simulink model "Car"  (R2023a)
settings: Solver=VariableStepAuto  StartTime=0.0  StopTime=1000  RelTol=1e-3
values from neighbouring files (symbols this model uses):
  AIR_DENSITY = 1.2    [Setup.m]
  FRONTAL_AREA = 1    [Setup.m]
  FULL_PACK_KWH = HV_PACK_VOLTAGE * HV_PACK_CAPACITY * UNIT_TO_KILO    (= 7.68)    [Setup.m]
  HV_PACK_VOLTAGE = 96    [Setup.m]
  INT_CURRENTS = CURRENT_DATA_ECO(1):0.0001:CURRENT_DATA_ECO(end)    [Setup.m]
  INT_TORQUES_ECO = interp1(CURRENT_DATA_ECO, TORQUES_DATA_ECO, INTERMEDIATE_VALUES,'spline')    [Setup.m]
  STARTING_KWH = FULL_PACK_KWH * (1 - 0.00)    (= 7.68)    [Setup.m]
  TARGET_SPEED = 25    [Setup.m]
  TOTAL_MASS = CAR_MASS + DRIVER_MASS    (= 282.996279643)    [Setup.m]
  UNIT_TO_KILO = 1 / 1000    (= 0.001)    [Setup.m]
undefined symbols (not defined in the file or in its folder): C_ROLLING_RESISTANCE, GRAVITY, MAX_TORQUE, WHEEL_RADIUS
libraries: slpidlib x1, simulink x1
settings Model: Creator=jcpetrie  LastModifiedBy=jcpetrie
settings ModelReferenceCC: EnableRefExpFcnMdlSchedulingChecks=on

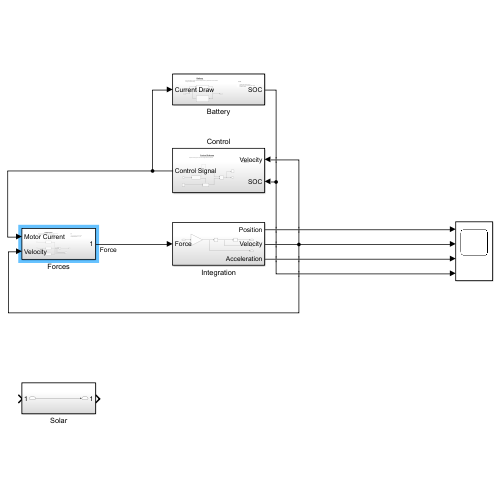
[thumbnail: Simulink's stored preview of the top-level diagram]
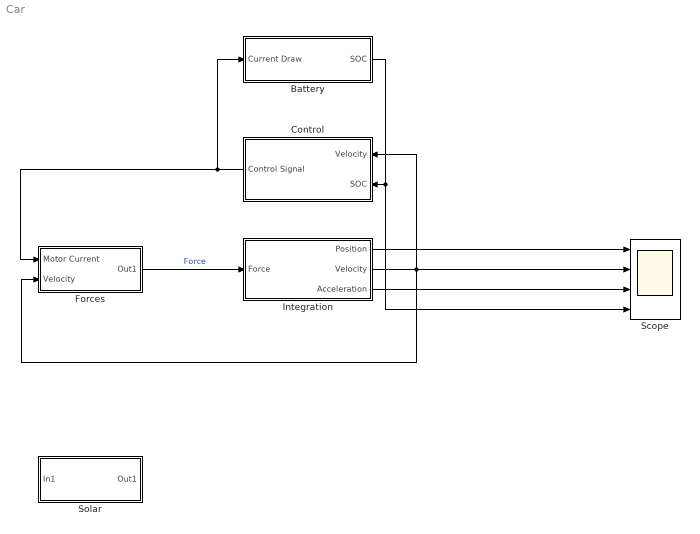
== system Car ==
  Battery : Subsystem
  Control : Subsystem
  Forces : Subsystem
  Integration : Subsystem
  Scope : Scope  NumInputPorts=4
  Solar : Subsystem
  wires:
  Control/1(Control Signal) -> Battery/1(Current Draw), Forces/1(Motor Current)
  Integration/2(Velocity) -> Forces/2(Velocity), Scope/2, Control/1(Velocity)
  Forces/1(Out1) -> Integration/1(Force)  "Force"
  Integration/1(Position) -> Scope/1
  Integration/3(Acceleration) -> Scope/3
  Battery/1(SOC) -> Scope/4, Control/2(SOC)

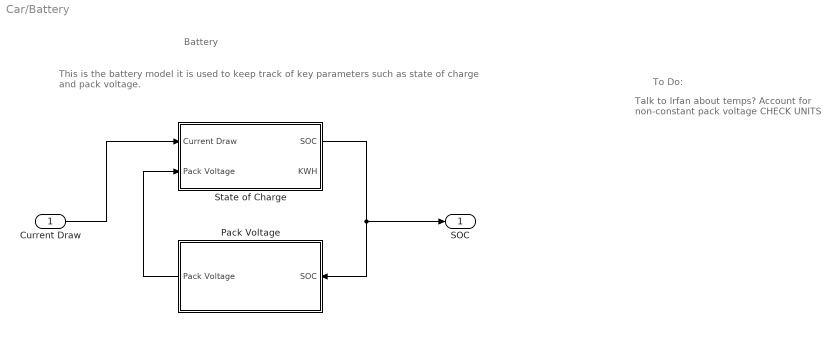
== system Car/Battery ==
  note: To Do:
  note: Battery
  note: This is the battery model it is used to keep track of key parameters such as state of charge and pack voltage.
  note: Talk to Irfan about temps?
      | Account for non-constant pack voltage
      | CHECK UNITS
  Current Draw : Inport
  Pack Voltage : Subsystem
  State of Charge : Subsystem
  SOC : Outport
  wires:
  Current Draw/1 -> State of Charge/1(Current Draw)
  State of Charge/1(SOC) -> Pack Voltage/1(SOC), SOC/1
  Pack Voltage/1(Pack Voltage) -> State of Charge/2(Pack Voltage)

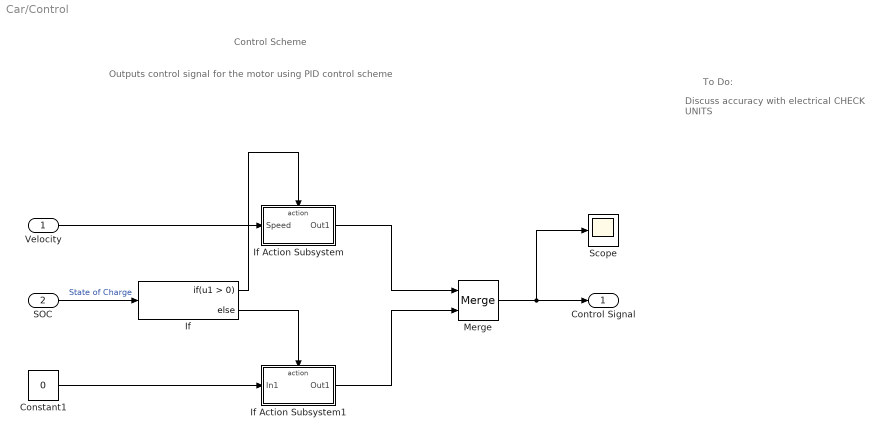
== system Car/Control ==
  note: Outputs control signal for the motor using PID control scheme
  note: To Do:
  note: Control Scheme
  note: Discuss accuracy with electrical
      | CHECK UNITS
  Velocity : Inport
  SOC : Inport  Port=2
  Constant1 : Constant  Value=0
  If : If
  If Action Subsystem : Subsystem  TreatAsAtomicUnit=on
  If Action Subsystem1 : Subsystem  TreatAsAtomicUnit=on
  Merge : Merge
  Scope : Scope
  Control Signal : Outport
  wires:
  Velocity/1 -> If Action Subsystem/1(Speed)
  SOC/1 -> If/1  "State of Charge"
  If/1 -> If Action Subsystem/Action
  If/2 -> If Action Subsystem1/Action
  Constant1/1 -> If Action Subsystem1/1(In1)
  If Action Subsystem/1(Out1) -> Merge/1
  If Action Subsystem1/1(Out1) -> Merge/2
  Merge/1 -> Scope/1, Control Signal/1

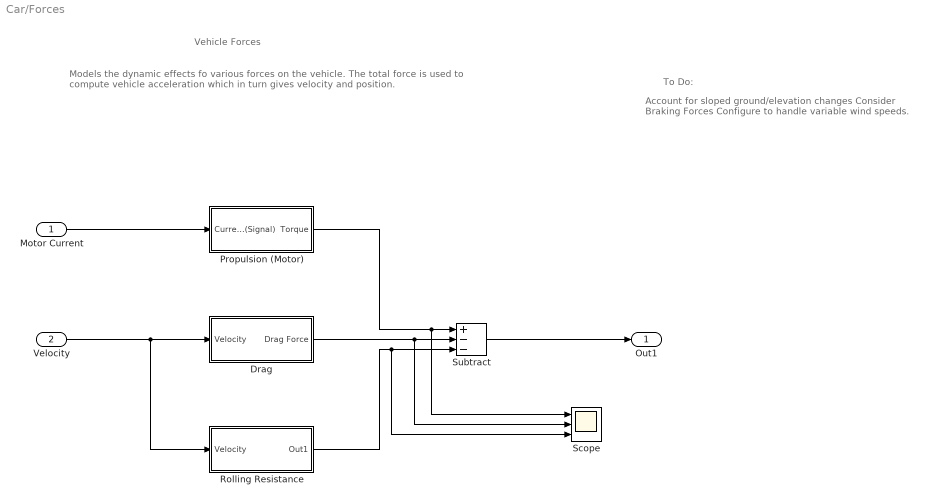
== system Car/Forces ==
  note: To Do:
  note: Vehicle Forces
  note: Models the dynamic effects fo various forces on the vehicle. The total force is used to compute vehicle acceleration which in turn gives velocity and position.
  note: Account for sloped ground/elevation changes
      | Consider Braking Forces
      | Configure to handle variable wind speeds.
  Motor Current : Inport
  Velocity : Inport  Port=2
  Drag : Subsystem
  Propulsion (Motor) : Subsystem
  Rolling Resistance : Subsystem
  Scope : Scope  NumInputPorts=3
  Subtract : Sum  Inputs=+--
  Out1 : Outport
  wires:
  Velocity/1 -> Rolling Resistance/1(Velocity), Drag/1(Velocity)
  Propulsion (Motor)/1(Torque) -> Scope/1, Subtract/1
  Drag/1(Drag Force) -> Scope/2, Subtract/2
  Rolling Resistance/1(Out1) -> Scope/3, Subtract/3
  Subtract/1 -> Out1/1
  Motor Current/1 -> Propulsion (Motor)/1(Current (Signal))

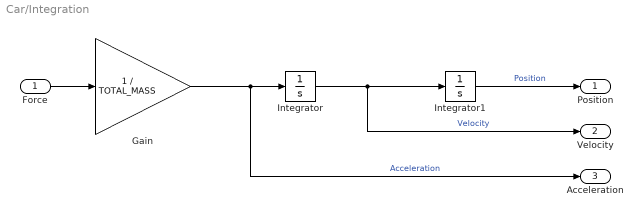
== system Car/Integration ==
  Force : Inport
  Gain : Gain  Gain=1 / TOTAL_MASS
  Integrator : Integrator
  Integrator1 : Integrator
  Position : Outport
  Velocity : Outport  Port=2
  Acceleration : Outport  Port=3
  wires:
  Gain/1 -> Acceleration/1, Integrator/1  "Acceleration"
  Integrator/1 -> Velocity/1, Integrator1/1  "Velocity"
  Force/1 -> Gain/1
  Integrator1/1 -> Position/1  "Position"

== system Car/Solar ==
  In1 : Inport
  Out1 : Outport
  wires:
  In1/1 -> Out1/1

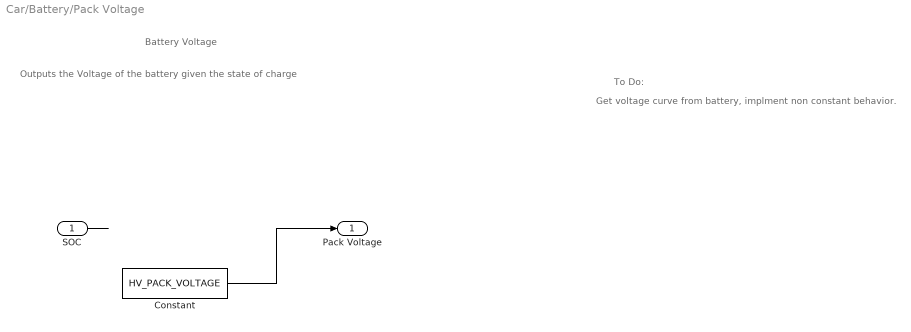
== system Car/Battery/Pack Voltage ==
  note: Battery Voltage
  note: Outputs the Voltage of the battery given the state of charge
  note: To Do:
  note: Get voltage curve from battery, implment non constant behavior.
  SOC : Inport
  Constant : Constant  Value=HV_PACK_VOLTAGE
  Pack Voltage : Outport
  wires:
  SOC/1 -> ?
  Constant/1 -> Pack Voltage/1

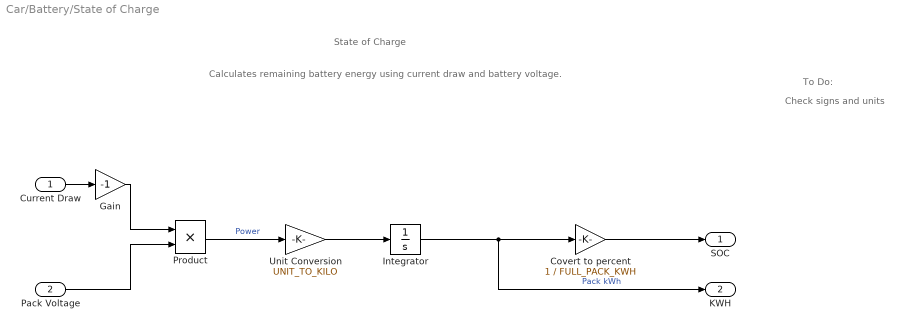
== system Car/Battery/State of Charge ==
  note: State of Charge
  note: Check signs and units
  note: To Do:
  note: Calculates remaining battery energy using current draw and battery voltage.
  Current Draw : Inport
  Pack Voltage : Inport  Port=2
  Covert to percent : Gain  Gain=1 / FULL_PACK_KWH
  Gain : Gain  Gain=-1
  Integrator : Integrator  InitialCondition=STARTING_KWH
  Product : Product  Inputs=**
  Unit Conversion : Gain  Gain=UNIT_TO_KILO
  SOC : Outport
  KWH : Outport  Port=2
  wires:
  Current Draw/1 -> Gain/1
  Integrator/1 -> KWH/1, Covert to percent/1  "Pack kWh"
  Covert to percent/1 -> SOC/1
  Pack Voltage/1 -> Product/2
  Product/1 -> Unit Conversion/1  "Power"
  Unit Conversion/1 -> Integrator/1
  Gain/1 -> Product/1

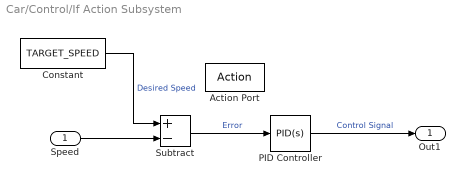
== system Car/Control/If Action Subsystem ==
  Speed : Inport
  Action Port : ActionPort  ActionPortLabel=if(u1 > 0)
  Constant : Constant  Value=TARGET_SPEED
  PID Controller : slpidlib/PID Controller  Controller=PID  Form=Parallel  TimeDomain=Continuous-time  UseExternalTs=off  SampleTime=-1  IntegratorMethod=Forward Euler  FilterMethod=Forward Euler  ControllerParametersSource=internal  P=2.5  I=0.1  UseKiTs=off  D=0  N=100  UseFilter=on  TunerSelectOption=Transfer Function Based (PID Tuner App)  InitialConditionSource=internal  InitialConditionForIntegrator=0  InitialConditionForFilter=0  DifferentiatorICPrevScaledInput=0  ExternalReset=none  TrackingMode=off  Kt=1  LimitOutput=off  SatLimitsSource=internal  UpperSaturationLimit=inf  LowerSaturationLimit=-inf  LinearizeAsGain=on  AntiWindupMode=none  Kb=1  LimitIntegrator=off  UpperIntegratorSaturationLimit=inf  LowerIntegratorSaturationLimit=-inf  POutMin=[]  POutMax=[]  IOutMin=[]  IOutMax=[]  DOutMin=[]  DOutMax=[]  NOutMin=[]  NOutMax=[]  SumOutMin=[]  SumOutMax=[]  SaturationOutMin=[]  SaturationOutMax=[]  PParamMin=[]  PParamMax=[]  IParamMin=[]  IParamMax=[]  DParamMin=[]  DParamMax=[]  NParamMin=[]  NParamMax=[]  KbParamMin=[]  KbParamMax=[]  KtParamMin=[]  KtParamMax=[]  KbOutMin=[]  KbOutMax=[]  KtOutMin=[]  KtOutMax=[]  IntegratorOutMin=[]  IntegratorOutMax=[]  FilterOutMin=[]  FilterOutMax=[]  SumI1OutMin=[]  SumI1OutMax=[]  SumI2OutMin=[]  SumI2OutMax=[]  SumI3OutMin=[]  SumI3OutMax=[]  SumI4OutMin=[]  SumI4OutMax=[]  SumDOutMin=[]  SumDOutMax=[]  DifferentiatorOutMin=[]  DifferentiatorOutMax=[]  FilterDiffOutCoefMin=[]  FilterDiffOutCoefMax=[]  ReciprocalOutMin=[]  ReciprocalOutMax=[]  SumDenOutMin=[]  SumDenOutMax=[]  SumNumOutMin=[]  SumNumOutMax=[]  DivideOutMin=[]  DivideOutMax=[]  UdiffTsProdOutMin=[]  UdiffTsProdOutMax=[]  NTsProdOutMin=[]  NTsProdOutMax=[]  UintegralTsProdOutMin=[]  UintegralTsProdOutMax=[]  UngainTsProdOutMin=[]  UngainTsProdOutMax=[]  ClampingZeroOutDataTypeStr=Inherit: Inherit via back propagation  ClampingZeroOutMin=[]  ClampingZeroOutMax=[]  FilterDenConstantOutDataTypeStr=Inherit: Inherit via back propagation  FilterDenConstantOutMin=[]  FilterDenConstantOutMax=[]  PCopyOutDataTypeStr=Inherit: Inherit via back propagation  PCopyOutMin=[]  PCopyOutMax=[]  NCopyOutDataTypeStr=Inherit: Inherit via back propagation  NCopyOutMin=[]  NCopyOutMax=[]  IntegratorContinuousStateAttributes=''  IntegratorStateMustResolveToSignalObject=off  IntegratorRTWStateStorageClass=Auto  FilterContinuousStateAttributes=''  FilterStateMustResolveToSignalObject=off  FilterRTWStateStorageClass=Auto  ParallelPVariant=InternalParameters  IdealPVariant=Disabled  IVariant=InternalParameters  DVariant=InternalParameters  IntegratorVariant=Continuous  SatVariant=Disabled  AWVariant=Passthrough  PCopyVariant=Disabled  TRVariant=Disabled  FdbkBlocksVariant=Forward  IdealPFdbkVariant=Disabled  SatFdbkVariant=Disabled  DerivativeFilterVariant=ContFilter  NVariant=InternalParameters  NCopyVariant=Disabled  FilterICVariant=InternalICsFilter  IntegratorICVariant=InternalICs  ExternalResetVariant=Disabled  TRSumVariant=Passthrough  SumFdbkVariant=Disabled  SumVariant=Sum_PID  TsampFilterVariant=InternalTs  TsampNgainVariant=Passthrough  TsampIntegralVariant=Disabled_SignalSpec  ExternalSaturationOutDataTypeStr=Inherit: Same as second input
  Subtract : Sum  Inputs=+-
  Out1 : Outport
  wires:
  Speed/1 -> Subtract/2
  PID Controller/1 -> Out1/1  "Control Signal"
  Constant/1 -> Subtract/1  "Desired Speed"
  Subtract/1 -> PID Controller/1  "Error"

== system Car/Control/If Action Subsystem1 ==
  In1 : Inport
  Action Port : ActionPort  ActionPortLabel=else
  Out1 : Outport
  wires:
  In1/1 -> Out1/1

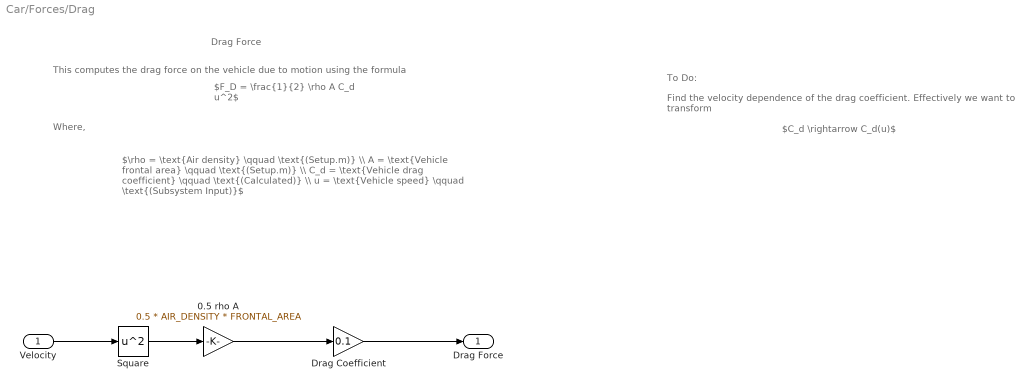
== system Car/Forces/Drag ==
  note: $C_d \rightarrow C_d(u)$
  note: Find the velocity dependence of the drag coefficient. Effectively we want to transform
  note: $\rho = \text{Air density} \qquad \text{(Setup.m)} \\ A = \text{Vehicle frontal area} \qquad \text{(Setup.m)} \\ C_d = \text{Vehicle drag coefficient} \qquad \text{(Calculated)} \\ u = \text{Vehicle speed} \qquad \text{(Subsystem Input)}$
  note: Where,
  note: $F_D = \frac{1}{2} \rho A C_d u^2$
  note: This computes the drag force on the vehicle due to motion using the formula
  note: To Do:
  note: Drag Force
  Velocity : Inport
  0.5 rho A : Gain  Gain=0.5 * AIR_DENSITY * FRONTAL_AREA
  Drag Coefficient : Gain  Gain=0.1
  Square : Math  Operator=square
  Drag Force : Outport
  wires:
  Velocity/1 -> Square/1
  Square/1 -> 0.5 rho A/1
  0.5 rho A/1 -> Drag Coefficient/1
  Drag Coefficient/1 -> Drag Force/1

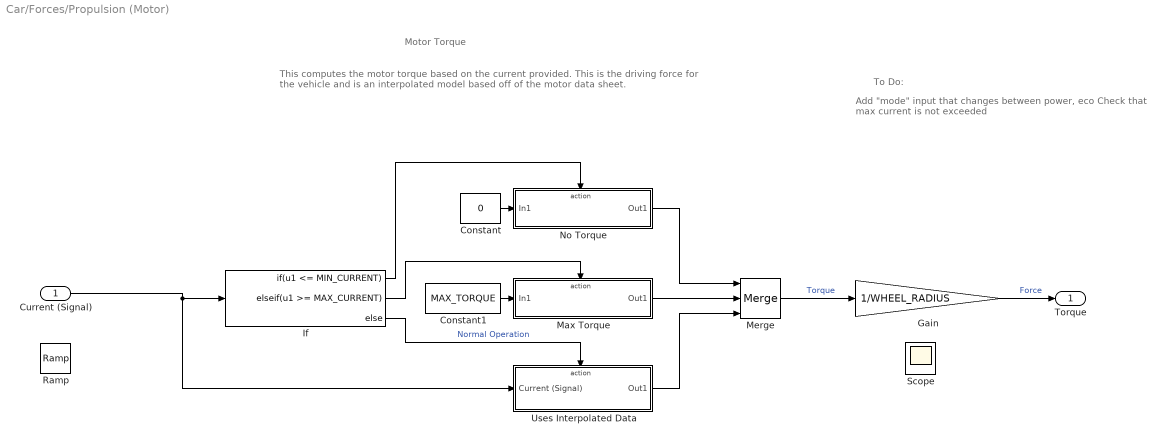
== system Car/Forces/Propulsion (Motor) ==
  note: Add "mode" input that changes between power, eco
      | Check that max current is not exceeded
  note: Motor Torque
  note: To Do:
  note: This computes the motor torque based on the current provided. This is the driving force for the vehicle and is an interpolated model based off of the motor data sheet.
  Current (Signal) : Inport
  Constant : Constant  Value=0
  Constant1 : Constant  Value=MAX_TORQUE
  Gain : Gain  Gain=1/WHEEL_RADIUS
  If : If  IfExpression=u1 <= MIN_CURRENT  ElseIfExpressions=u1 >= MAX_CURRENT
  Max Torque : Subsystem  TreatAsAtomicUnit=on
  Merge : Merge  Inputs=3
  No Torque : Subsystem  TreatAsAtomicUnit=on
  Ramp : simulink/Sources/Ramp  slope=1  start=0  InitialOutput=-1
  Scope : Scope
  Uses Interpolated Data : Subsystem  TreatAsAtomicUnit=on
  Torque : Outport
  wires:
  Current (Signal)/1 -> Uses Interpolated Data/1(Current (Signal)), If/1
  Constant/1 -> No Torque/1(In1)
  If/1 -> No Torque/Action
  If/2 -> Max Torque/Action
  Uses Interpolated Data/1(Out1) -> Merge/3
  No Torque/1(Out1) -> Merge/1
  Merge/1 -> Gain/1  "Torque"
  If/3 -> Uses Interpolated Data/Action  "Normal Operation"
  Constant1/1 -> Max Torque/1(In1)
  Max Torque/1(Out1) -> Merge/2
  Gain/1 -> Torque/1  "Force"

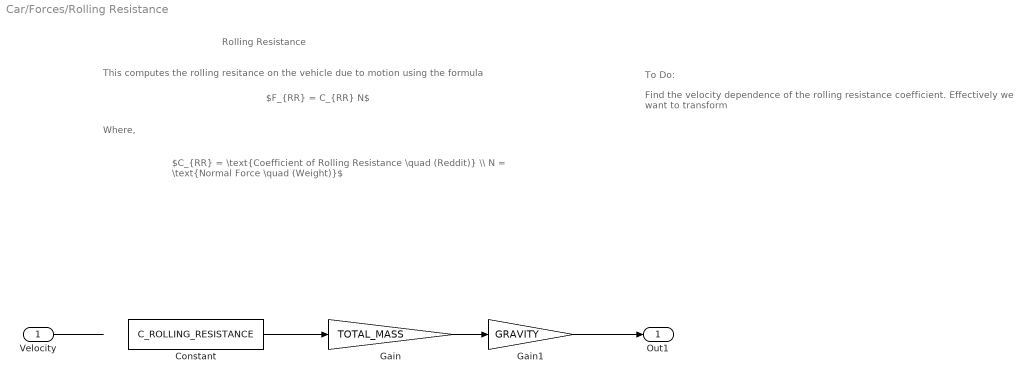
== system Car/Forces/Rolling Resistance ==
  note: This computes the rolling resitance on the vehicle due to motion using the formula
  note: To Do:
  note: $C_{RR} = \text{Coefficient of Rolling Resistance \quad (Reddit)} \\ N = \text{Normal Force \quad (Weight)}$
  note: Where,
  note: Find the velocity dependence of the rolling resistance coefficient. Effectively we want to transform
  note: Rolling Resistance
  note: $F_{RR} = C_{RR} N$
  Velocity : Inport
  Constant : Constant  Value=C_ROLLING_RESISTANCE
  Gain : Gain  Gain=TOTAL_MASS
  Gain1 : Gain  Gain=GRAVITY
  Out1 : Outport
  wires:
  Velocity/1 -> ?
  Gain/1 -> Gain1/1
  Constant/1 -> Gain/1
  Gain1/1 -> Out1/1

== system Car/Forces/Propulsion (Motor)/Max Torque ==
  In1 : Inport
  Action Port : ActionPort  ActionPortLabel=elseif(u1 >= MAX_CURRENT)
  Out1 : Outport
  wires:
  In1/1 -> Out1/1

== system Car/Forces/Propulsion (Motor)/No Torque ==
  In1 : Inport
  Action Port : ActionPort  ActionPortLabel=if(u1 <= MIN_CURRENT)
  Out1 : Outport
  wires:
  In1/1 -> Out1/1

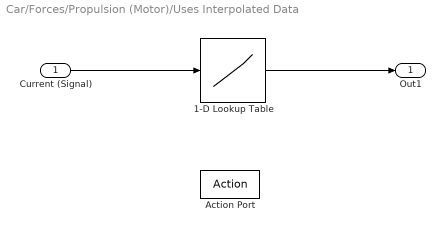
== system Car/Forces/Propulsion (Motor)/Uses Interpolated Data ==
  Current (Signal) : Inport
  Action Port : ActionPort  ActionPortLabel=else
  1-D Lookup Table : Lookup_n-D  NumberOfTableDimensions=1  LookupTableObject=''  BreakpointsForDimension1=INT_CURRENTS  BreakpointsForDimension1FirstPoint=10  BreakpointsForDimension2FirstPoint=10  BreakpointsForDimension1Spacing=12  BreakpointsForDimension2Spacing=12  Table=INT_TORQUES_ECO  DiagnosticForOutOfRangeInput=Warning  InternalRulePriority=Speed  RndMeth=Simplest
  Out1 : Outport
  wires:
  Current (Signal)/1 -> 1-D Lookup Table/1
  1-D Lookup Table/1 -> Out1/1
